simulink model "week3_p_cruise_control"  (R2025b)
settings: Solver=VariableStepAuto  StartTime=0.0  StopTime=100  RelTol=1e-3
undefined symbols (not defined in the file): A_front, Cd, Cr, g, m, rho, v0
settings Model: Creator=legob  LastModifiedBy=legob

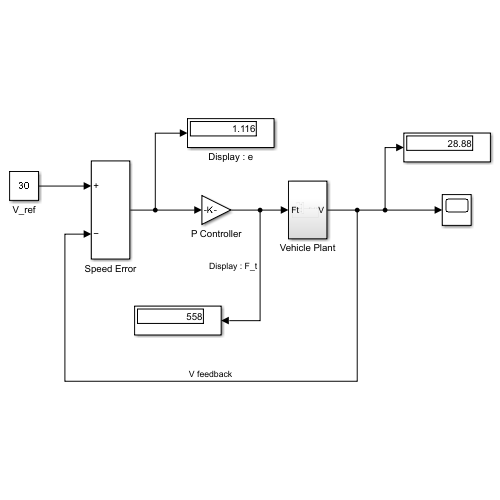
[thumbnail: Simulink's stored preview of the top-level diagram]
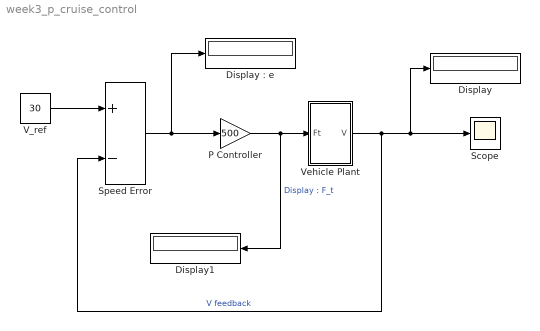
== system week3_p_cruise_control ==
  Display : Display
  "Display : e" : Display
  Display1 : Display
  P Controller : Gain  Gain=500
  Scope : Scope
      settings: ActiveDisplayYMinimum=-209.12652721389364  ActiveDisplayYMaximum=177.61826373731512
  Speed Error : Sum  Inputs=+-
  V_ref : Constant  Value=30
  Vehicle Plant : Subsystem
  wires:
  Vehicle Plant/1(V) -> Speed Error/2, Display/1, Scope/1  "V feedback"
  V_ref/1 -> Speed Error/1
  Speed Error/1 -> "Display : e"/1, P Controller/1
  P Controller/1 -> Display1/1, Vehicle Plant/1(Ft)  "Display : F_t"

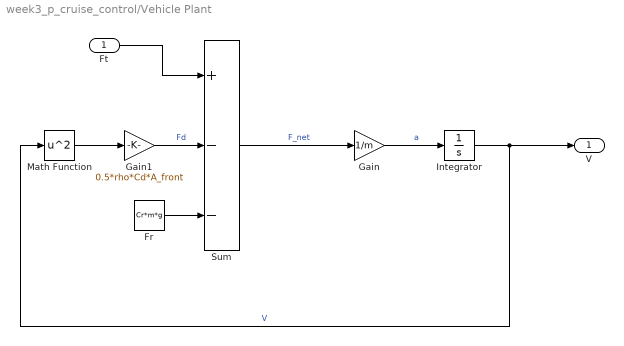
== system week3_p_cruise_control/Vehicle Plant ==
  Ft : Inport
  Fr : Constant  Value=Cr*m*g
  Gain : Gain  Gain=1/m
  Gain1 : Gain  Gain=0.5*rho*Cd*A_front
  Integrator : Integrator  InitialCondition=v0
  Math Function : Math  Operator=square
  Sum : Sum  Inputs=+--
  V : Outport
  wires:
  Fr/1 -> Sum/3
  Integrator/1 -> V/1, Math Function/1  "V"
  Sum/1 -> Gain/1  "F_net"
  Gain/1 -> Integrator/1  "a"
  Ft/1 -> Sum/1
  Gain1/1 -> Sum/2  "Fd"
  Math Function/1 -> Gain1/1
